simulink model "gm_uz_pmsm_model_nonlinear"  (R2023a)
settings: Solver=FixedStepAuto  StartTime=0.0  StopTime=0.5  RelTol=1e-3
PreLoadFcn:
  | uz_pmsm_model_init_parameter
PostLoadFcn:
  | % Import the data from Excel for a lookup table
  | FluxMapData = readtable('C:\Users\Philipp\ultrazohm\ultrazohm_sw\ip_cores\uz_pmsm_model\FluxMapData_2023-05-26_13-07-57.csv');
  | % Row indices for lookup table
  | d_current_in_d_axis = FluxMapData(8:27,1:end);
  | % Column indices for lookup table
  | q_current_in_d_axis = FluxMapData(29:48,1:end);
  | % Output values for lookup table
  | d_Flux_d_axis = FluxMapData(50:69,1:end);
undefined symbols (not defined in the file or in its folder): d_current_d_Flux, d_current_q_Flux, Flux_d, Flux_q, friction_coefficient, inertia, k_i_d, k_p_d, k_p_q, L_d, L_q, Ldd, Ldq, Lqd, Lqq, polepair, psi_pm, q_current_d_Flux, q_current_q_Flux, R_1, setpoint_step, simulate_mechanical, simulate_open_loop, static_friction_torque
libraries: hdlmdlgenlib x8, slpidlib x2
(part 2 of 2)

== system gm_uz_pmsm_model_nonlinear/uz_pmsm_model_nonlinear/Product91 ==
  In1 : Inport
  In2 : Inport  Port=2
  Product91 : Product  Inputs=**  OutDataTypeStr=double  SampleTime=1e-08
  Product91_pd1 : Delay  DelayLength=6
  Out1 : Outport
  wires:
  In1/1 -> Product91/1
  In2/1 -> Product91/2
  Product91/1 -> Product91_pd1/1
  Product91_pd1/1 -> Out1/1

== system gm_uz_pmsm_model_nonlinear/uz_pmsm_model_nonlinear/Sign1 ==
  In1 : Inport
  Sign1 : Signum  SampleTime=1e-08
  Out1 : Outport
  wires:
  In1/1 -> Sign1/1
  Sign1/1 -> Out1/1

== system gm_uz_pmsm_model_nonlinear/uz_pmsm_model_nonlinear/Sum ==
  In1 : Inport
  In2 : Inport  Port=2
  Sum : Sum  Inputs=+-  OutDataTypeStr=double  SampleTime=1e-08
  Sum_pd1 : Delay  DelayLength=6
  Out1 : Outport
  wires:
  In1/1 -> Sum/1
  In2/1 -> Sum/2
  Sum/1 -> Sum_pd1/1
  Sum_pd1/1 -> Out1/1

== system gm_uz_pmsm_model_nonlinear/uz_pmsm_model_nonlinear/Sum1 ==
  In1 : Inport
  In2 : Inport  Port=2
  Sum1 : Sum  Inputs=+-  OutDataTypeStr=double  SampleTime=1e-08
  Sum1_pd1 : Delay  DelayLength=6
  Out1 : Outport
  wires:
  In1/1 -> Sum1/1
  In2/1 -> Sum1/2
  Sum1/1 -> Sum1_pd1/1
  Sum1_pd1/1 -> Out1/1

== system gm_uz_pmsm_model_nonlinear/uz_pmsm_model_nonlinear/Sum3 ==
  In1 : Inport
  In2 : Inport  Port=2
  Sum3 : Sum  OutDataTypeStr=double  SampleTime=1e-08
  Sum3_pd1 : Delay  DelayLength=6
  Out1 : Outport
  wires:
  In1/1 -> Sum3/1
  In2/1 -> Sum3/2
  Sum3/1 -> Sum3_pd1/1
  Sum3_pd1/1 -> Out1/1

== system gm_uz_pmsm_model_nonlinear/uz_pmsm_model_nonlinear/Sum31 ==
  In1 : Inport
  In2 : Inport  Port=2
  Sum31 : Sum  Inputs=+-  OutDataTypeStr=double  SampleTime=1e-08
  Sum31_pd1 : Delay  DelayLength=6
  Out1 : Outport
  wires:
  In1/1 -> Sum31/1
  In2/1 -> Sum31/2
  Sum31/1 -> Sum31_pd1/1
  Sum31_pd1/1 -> Out1/1

== system gm_uz_pmsm_model_nonlinear/uz_pmsm_model_nonlinear/Sum3_stage2 ==
  In1 : Inport
  In2 : Inport  Port=2
  Sum3_stage2 : Sum  Inputs=+-  OutDataTypeStr=double  SampleTime=1e-08
  Sum3_stage2_pd1 : Delay  DelayLength=6
  Out1 : Outport
  wires:
  In1/1 -> Sum3_stage2/1
  In2/1 -> Sum3_stage2/2
  Sum3_stage2/1 -> Sum3_stage2_pd1/1
  Sum3_stage2_pd1/1 -> Out1/1

== system gm_uz_pmsm_model_nonlinear/uz_pmsm_model_nonlinear/Sum3_stage3 ==
  In1 : Inport
  In2 : Inport  Port=2
  Sum3_stage3 : Sum  Inputs=+-  OutDataTypeStr=double  SampleTime=1e-08
  Sum3_stage3_pd1 : Delay  DelayLength=6
  Out1 : Outport
  wires:
  In1/1 -> Sum3_stage3/1
  In2/1 -> Sum3_stage3/2
  Sum3_stage3/1 -> Sum3_stage3_pd1/1
  Sum3_stage3_pd1/1 -> Out1/1

== system gm_uz_pmsm_model_nonlinear/uz_pmsm_model_nonlinear/Sum3_stage4 ==
  In1 : Inport
  In2 : Inport  Port=2
  Sum3_stage4 : Sum  OutDataTypeStr=double  SampleTime=1e-08
  Sum3_stage4_pd1 : Delay  DelayLength=6
  Out1 : Outport
  wires:
  In1/1 -> Sum3_stage4/1
  In2/1 -> Sum3_stage4/2
  Sum3_stage4/1 -> Sum3_stage4_pd1/1
  Sum3_stage4_pd1/1 -> Out1/1

== system gm_uz_pmsm_model_nonlinear/uz_pmsm_model_nonlinear/Sum4_stage2 ==
  In1 : Inport
  In2 : Inport  Port=2
  Sum4_stage2 : Sum  Inputs=+-  OutDataTypeStr=double  SampleTime=1e-08
  Sum4_stage2_pd1 : Delay  DelayLength=6
  Out1 : Outport
  wires:
  In1/1 -> Sum4_stage2/1
  In2/1 -> Sum4_stage2/2
  Sum4_stage2/1 -> Sum4_stage2_pd1/1
  Sum4_stage2_pd1/1 -> Out1/1

== system gm_uz_pmsm_model_nonlinear/uz_pmsm_model_nonlinear/Sum4_stage3 ==
  In1 : Inport
  In2 : Inport  Port=2
  Sum4_stage3 : Sum  Inputs=+-  OutDataTypeStr=double  SampleTime=1e-08
  Sum4_stage3_pd1 : Delay  DelayLength=6
  Out1 : Outport
  wires:
  In1/1 -> Sum4_stage3/1
  In2/1 -> Sum4_stage3/2
  Sum4_stage3/1 -> Sum4_stage3_pd1/1
  Sum4_stage3_pd1/1 -> Out1/1

== system gm_uz_pmsm_model_nonlinear/uz_pmsm_model_nonlinear/Sum4_stage4 ==
  In1 : Inport
  In2 : Inport  Port=2
  Sum4_stage4 : Sum  Inputs=+-  OutDataTypeStr=double  SampleTime=1e-08
  Sum4_stage4_pd1 : Delay  DelayLength=6
  Out1 : Outport
  wires:
  In1/1 -> Sum4_stage4/1
  In2/1 -> Sum4_stage4/2
  Sum4_stage4/1 -> Sum4_stage4_pd1/1
  Sum4_stage4_pd1/1 -> Out1/1

== system gm_uz_pmsm_model_nonlinear/uz_pmsm_model_nonlinear/Sum5 ==
  In1 : Inport
  In2 : Inport  Port=2
  Sum5 : Sum  OutDataTypeStr=double  SampleTime=1e-08
  Sum5_pd1 : Delay  DelayLength=6
  Out1 : Outport
  wires:
  In1/1 -> Sum5/1
  In2/1 -> Sum5/2
  Sum5/1 -> Sum5_pd1/1
  Sum5_pd1/1 -> Out1/1

== system gm_uz_pmsm_model_nonlinear/uz_pmsm_model_nonlinear/Sum51 ==
  In1 : Inport
  In2 : Inport  Port=2
  Sum51 : Sum  OutDataTypeStr=double  SampleTime=1e-08
  Sum51_pd1 : Delay  DelayLength=6
  Out1 : Outport
  wires:
  In1/1 -> Sum51/1
  In2/1 -> Sum51/2
  Sum51/1 -> Sum51_pd1/1
  Sum51_pd1/1 -> Out1/1

== system gm_uz_pmsm_model_nonlinear/uz_pmsm_model_nonlinear/Sum52 ==
  In1 : Inport
  In2 : Inport  Port=2
  Sum52 : Sum  OutDataTypeStr=double  SampleTime=1e-08
  Sum52_pd1 : Delay  DelayLength=6
  Out1 : Outport
  wires:
  In1/1 -> Sum52/1
  In2/1 -> Sum52/2
  Sum52/1 -> Sum52_pd1/1
  Sum52_pd1/1 -> Out1/1
